simulink model "LeftTurn"  (R2023b)
settings: Solver=FixedStepAuto  StartTime=0.0  StopTime=inf  RelTol=1e-3
undefined symbols (not defined in the file or in its folder): DiscIntNeverNeededParam
libraries: arduinolib x14, simulink x12, mobileRoboticsTrainingLib x1, arduinosensorlib x1
settings Model: ExtModeTrigDuration=2  Creator=cameronclark  LastModifiedBy=cameronclark
settings OptimizationCC: EnhancedBackFolding=on  PassReuseOutputArgsAs=Individual arguments  ZeroExternalMemoryAtStartup=off  ZeroInternalMemoryAtStartup=off  MaxStackSize=64  OptimizeBlockOrder=speed  DifferentSizesBufferReuse=on  OptimizationCustomize=off  EfficientTunableParamExpr=on
settings DebuggingCC: ParameterTunabilityLossMsg=error
settings HardwareCC: ProdBitPerPointer=32  ProdBitPerSizeT=32  ProdBitPerPtrDiffT=32  ProdLargestAtomicInteger=Long  ProdLargestAtomicFloat=Double  ProdWordSize=32  ProdHWDeviceType=ARM Compatible->ARM Cortex  UseEmbeddedCoderFeatures=off  UseSimulinkCoderFeatures=off
settings SFSimCC: MATLABDynamicMemAlloc=off
settings RTWCC: Description=Embedded Coder  SystemTargetFile=ert.tlc  HardwareBoard=Arduino Nano 33 IoT  TemplateMakefile=ert_default_tmf  Toolchain=Arduino ARM  BuildConfiguration=Faster Runs
settings CodeAppCC: ForceParamTrailComments=on  IgnoreCustomStorageClasses=off  OperatorAnnotations=on  SimulinkDataObjDesc=on  SFDataObjDesc=on  InsertBlockDesc=on
settings ERTTargetCC: SupportContinuousTime=on  SupportNonInlinedSFcns=on  SupportVariableSizeSignals=on  ExtModeTransport=3  ExtModeStaticAlloc=on  ExtModeAutomaticAllocSize=off  ExtModeStaticAllocSize=8192  ExtModeMexFile=ext_xcp  ExtModeIntrfLevel=Level2 - Open

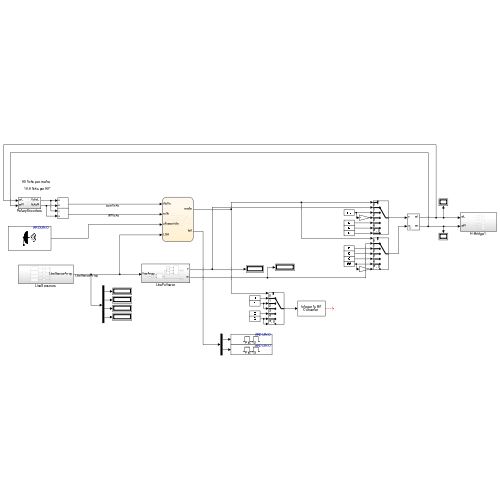
[thumbnail: Simulink's stored preview of the top-level diagram]
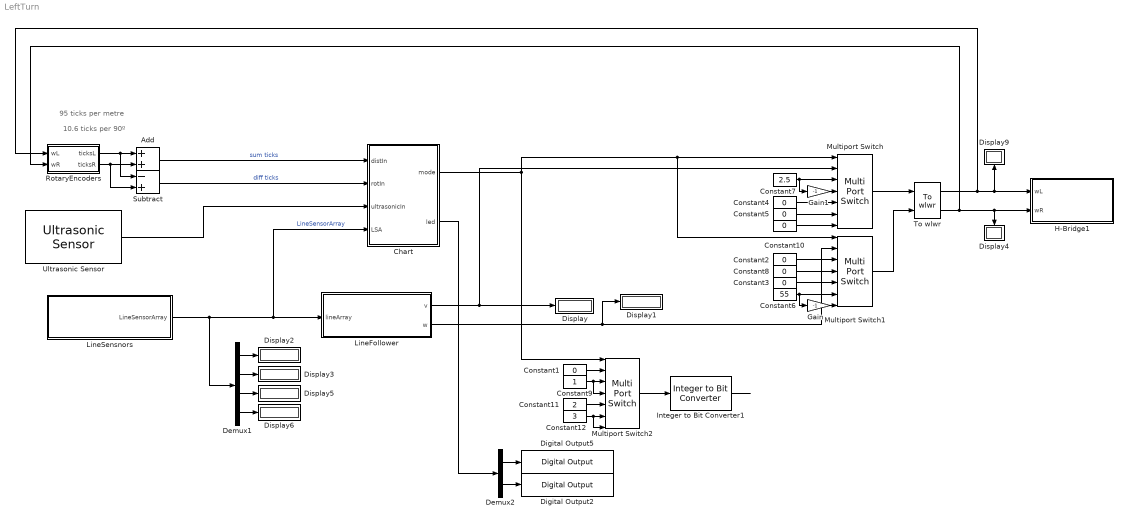
== system LeftTurn ==
  note: 10.6 ticks per 90º
  note: 95 ticks per metre
  Add : Sum
  Chart : Stateflow chart  TreatAsAtomicUnit=on
  Constant{1..5,8,10} (7 alike) : Constant  Value=0
  Constant11 : Constant  Value=2
  Constant12 : Constant  Value=3
  Constant6 : Constant  Value=55
  Constant7 : Constant  Value=2.5
  Constant9 : Constant
  Demux1 : Demux
  Demux2 : Demux  Outputs=2
  Digital Output2 : arduinolib/Digital Output  pinNumber=13  Direction=output  blockPlatform=arduino
  Digital Output5 : arduinolib/Digital Output  pinNumber=12  Direction=output  blockPlatform=arduino
  Display{,1..6,9} (8 alike) : Display
  Gain : Gain  Gain=-1
  Gain1 : Gain  Gain=-1
  H-Bridge1 : Subsystem
  Integer to Bit Converter1 : simulink/Logic and Bit Operations/Integer to Bit Converter  nbits=2  signedInputValues=Unsigned  bitOrder=MSB first  outDtype=Inherit via internal rule
  LineFollower : Subsystem
  LineSensnors : Subsystem
  Multiport Switch : MultiPortSwitch  DataPortOrder=Zero-based contiguous  Inputs=6  DataPortIndices={0,1,3,4}  zeroidx=on  SaturateOnIntegerOverflow=off
  Multiport Switch1 : MultiPortSwitch  DataPortOrder=Zero-based contiguous  Inputs=6  DataPortIndices={0,1,3,4}  zeroidx=on  SaturateOnIntegerOverflow=off  InputSameDT=off
  Multiport Switch2 : MultiPortSwitch  DataPortOrder=Zero-based contiguous  Inputs=6  DataPortIndices={0,1,3,4}  zeroidx=on  SaturateOnIntegerOverflow=off  InputSameDT=off
  RotaryEncoders : Subsystem
  Subtract : Sum  Inputs=-+
  To wlwr : mobileRoboticsTrainingLib/To wlwr  axleLength=0.1  wheelR=0.05
      link override change parameters: Gain=[1 -axleLength/2;1 axleLength/2]
  Ultrasonic Sensor : arduinosensorlib/Ultrasonic Sensor  NumSignalPins=2  TrigPin=8  EchoPin=11  SignalPin=3  SampleTime_=0.1  blockPlatform=ARDUINO
  wires:
  Ultrasonic Sensor/1 -> Chart/3(ultrasonicIn)
  LineFollower/1(v) -> Multiport Switch/2, Display/1
  Multiport Switch/1 -> To wlwr/1
  RotaryEncoders/2(ticksR) -> Subtract/2, Add/2
  Subtract/1 -> Chart/2(rotIn)  "diff ticks"
  Add/1 -> Chart/1(distIn)  "sum ticks"
  Constant7/1 -> Gain1/1, Multiport Switch/3
  LineFollower/2(w) -> Multiport Switch1/2, Display1/1
  RotaryEncoders/1(ticksL) -> Subtract/1, Add/1
  Constant5/1 -> Multiport Switch/6
  Constant2/1 -> Multiport Switch1/3
  Constant3/1 -> Multiport Switch1/5
  Multiport Switch1/1 -> To wlwr/2
  Constant4/1 -> Multiport Switch/5
  LineSensnors/1(LineSensorArray) -> Demux1/1, LineFollower/1(lineArray), Chart/4(LSA)  "LineSensorArray"
  Chart/1(mode) -> Multiport Switch2/1, Multiport Switch1/1, Multiport Switch/1
  Constant8/1 -> Multiport Switch1/4
  Constant10/1 -> Multiport Switch/7
  Demux1/1 -> Display2/1
  Demux1/2 -> Display3/1
  Demux1/3 -> Display5/1
  Demux1/4 -> Display6/1
  To wlwr/2 -> RotaryEncoders/2(wR), H-Bridge1/2(wR), Display4/1
  To wlwr/1 -> RotaryEncoders/1(wL), H-Bridge1/1(wL), Display9/1
  Constant6/1 -> Gain/1, Multiport Switch1/6
  Gain/1 -> Multiport Switch1/7
  Gain1/1 -> Multiport Switch/4
  Integer to Bit Converter1/1 -> ?
  Multiport Switch2/1 -> Integer to Bit Converter1/1
  Constant1/1 -> Multiport Switch2/2
  Constant9/1 -> Multiport Switch2/4, Multiport Switch2/3
  Constant11/1 -> Multiport Switch2/5
  Constant12/1 -> Multiport Switch2/7, Multiport Switch2/6
  Demux2/1 -> Digital Output5/1
  Demux2/2 -> Digital Output2/1
  Chart/2(led) -> Demux2/1

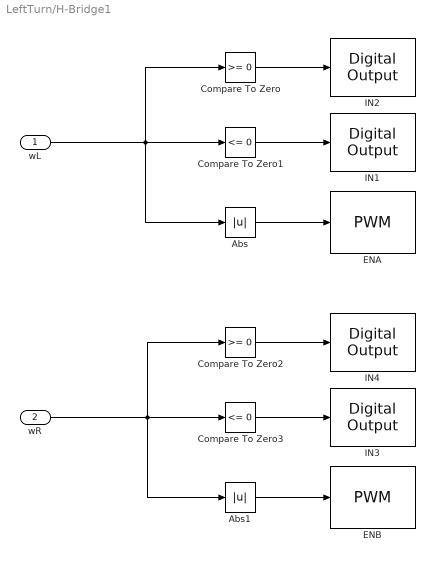
== system LeftTurn/H-Bridge1 ==
  wL : Inport
  wR : Inport  Port=2
  Abs : Abs  SaturateOnIntegerOverflow=off
  Abs1 : Abs  SaturateOnIntegerOverflow=off
  Compare To Zero : simulink/Logic and Bit Operations/Compare To Zero  relop=>=  OutDataTypeStr=boolean
  Compare To Zero1 : simulink/Logic and Bit Operations/Compare To Zero  relop=<=  OutDataTypeStr=boolean
  Compare To Zero2 : simulink/Logic and Bit Operations/Compare To Zero  relop=>=  OutDataTypeStr=boolean
  Compare To Zero3 : simulink/Logic and Bit Operations/Compare To Zero  relop=<=  OutDataTypeStr=boolean
  ENA : arduinolib/PWM  pinNumber=4  frequencyType=Default  desiredFrequency=490.2  achievableFrequency=490.2
  ENB : arduinolib/PWM  pinNumber=5  frequencyType=Default  desiredFrequency=490.2  achievableFrequency=490.2
  IN1 : arduinolib/Digital Output  pinNumber=2  Direction=output  blockPlatform=arduino
  IN2 : arduinolib/Digital Output  pinNumber=3  Direction=output  blockPlatform=arduino
  IN3 : arduinolib/Digital Output  pinNumber=6  Direction=output  blockPlatform=arduino
  IN4 : arduinolib/Digital Output  pinNumber=7  Direction=output  blockPlatform=arduino
  wires:
  Compare To Zero1/1 -> IN1/1
  Compare To Zero/1 -> IN2/1
  Abs1/1 -> ENB/1
  Compare To Zero3/1 -> IN3/1
  Compare To Zero2/1 -> IN4/1
  wL/1 -> Compare To Zero/1, Compare To Zero1/1, Abs/1
  Abs/1 -> ENA/1
  wR/1 -> Compare To Zero2/1, Compare To Zero3/1, Abs1/1

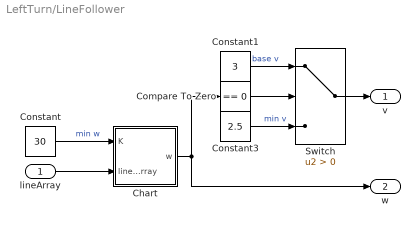
== system LeftTurn/LineFollower ==
  lineArray : Inport
  Chart : Stateflow chart  TreatAsAtomicUnit=on
  Compare To Zero : simulink/Logic and Bit Operations/Compare To Zero  relop===  OutDataTypeStr=boolean
  Constant : Constant  Value=30
  Constant1 : Constant  Value=3
  Constant3 : Constant  Value=2.5
  Switch : Switch  Criteria=u2 > Threshold  SaturateOnIntegerOverflow=off  InputSameDT=off
  v : Outport
  w : Outport  Port=2
  wires:
  Constant1/1 -> Switch/1  "base v"
  Chart/1(w) -> Compare To Zero/1, w/1
  Constant3/1 -> Switch/3  "min v"
  Switch/1 -> v/1
  lineArray/1 -> Chart/2(lineArray)
  Compare To Zero/1 -> Switch/2
  Constant/1 -> Chart/1(K)  "min w"

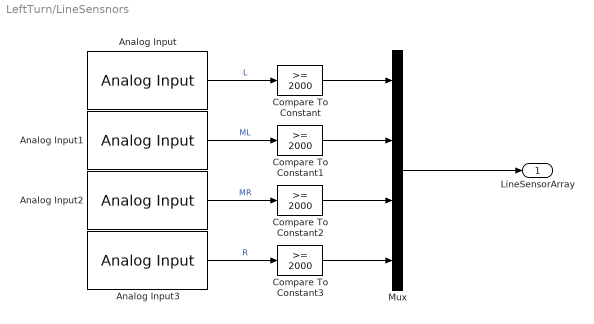
== system LeftTurn/LineSensnors ==
  Analog Input : arduinolib/Analog Input  pinNumber=7  ReadResultsOnly=off  ConversionTriggerSource=Software  ExternalTriggerType=uint32( 0 )  OutputDataType=uint16  EnableConversionCompleteNotify=off  EnableOuputStatus=off  SampleTime=-1  blockPlatform=arduino
  Analog Input1 : arduinolib/Analog Input  pinNumber=6  ReadResultsOnly=off  ConversionTriggerSource=Software  ExternalTriggerType=uint32( 0 )  OutputDataType=uint16  EnableConversionCompleteNotify=off  EnableOuputStatus=off  SampleTime=-1  blockPlatform=arduino
  Analog Input2 : arduinolib/Analog Input  pinNumber=3  ReadResultsOnly=off  ConversionTriggerSource=Software  ExternalTriggerType=uint32( 0 )  OutputDataType=uint16  EnableConversionCompleteNotify=off  EnableOuputStatus=off  SampleTime=-1  blockPlatform=arduino
  Analog Input3 : arduinolib/Analog Input  pinNumber=2  ReadResultsOnly=off  ConversionTriggerSource=Software  ExternalTriggerType=uint32( 0 )  OutputDataType=uint16  EnableConversionCompleteNotify=off  EnableOuputStatus=off  SampleTime=-1  blockPlatform=arduino
  Compare To Constant{,1..3} (4 alike) : simulink/Logic and Bit Operations/Compare To Constant  relop=>=  const=2000  OutDataTypeStr=boolean
  Mux : Mux
  LineSensorArray : Outport
  wires:
  Mux/1 -> LineSensorArray/1
  Analog Input/1 -> Compare To Constant/1  "L"
  Analog Input1/1 -> Compare To Constant1/1  "ML"
  Analog Input2/1 -> Compare To Constant2/1  "MR"
  Analog Input3/1 -> Compare To Constant3/1  "R"
  Compare To Constant/1 -> Mux/1
  Compare To Constant1/1 -> Mux/2
  Compare To Constant2/1 -> Mux/3
  Compare To Constant3/1 -> Mux/4

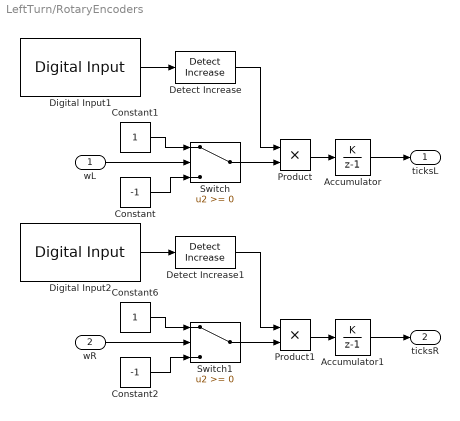
== system LeftTurn/RotaryEncoders ==
  wL : Inport
  wR : Inport  Port=2
  Accumulator : DiscreteIntegrator  IntegratorMethod=Accumulation: Forward Euler  SampleTime=-1  ICPrevOutput=DiscIntNeverNeededParam  ICPrevScaledInput=DiscIntNeverNeededParam
  Accumulator1 : DiscreteIntegrator  IntegratorMethod=Accumulation: Forward Euler  SampleTime=-1  ICPrevOutput=DiscIntNeverNeededParam  ICPrevScaledInput=DiscIntNeverNeededParam
  Constant : Constant  Value=-1
  Constant1 : Constant
  Constant2 : Constant  Value=-1
  Constant6 : Constant
  Detect Increase : simulink/Logic and Bit Operations/Detect Increase  vinit=0.0  OutDataTypeStr=boolean
  Detect Increase1 : simulink/Logic and Bit Operations/Detect Increase  vinit=0.0  OutDataTypeStr=boolean
  Digital Input1 : arduinolib/Digital Input  pinNumber=9  mode=Default  Direction=input  SampleTime=0.1  blockPlatform=arduino
  Digital Input2 : arduinolib/Digital Input  pinNumber=10  mode=Default  Direction=input  SampleTime=0.1  blockPlatform=arduino
  Product : Product
  Product1 : Product
  Switch : Switch  SaturateOnIntegerOverflow=off  InputSameDT=off
  Switch1 : Switch  SaturateOnIntegerOverflow=off  InputSameDT=off
  ticksL : Outport
  ticksR : Outport  Port=2
  wires:
  wL/1 -> Switch/2
  Constant1/1 -> Switch/1
  Constant/1 -> Switch/3
  Digital Input1/1 -> Detect Increase/1
  Switch/1 -> Product/2
  Accumulator/1 -> ticksL/1
  wR/1 -> Switch1/2
  Constant6/1 -> Switch1/1
  Constant2/1 -> Switch1/3
  Accumulator1/1 -> ticksR/1
  Switch1/1 -> Product1/2
  Product/1 -> Accumulator/1
  Detect Increase/1 -> Product/1
  Detect Increase1/1 -> Product1/1
  Digital Input2/1 -> Detect Increase1/1
  Product1/1 -> Accumulator1/1

== stateflow chart LeftTurn/LineFollower/Chart ==
  state ComputeW
    %code for the line array
    during:
    w = K*(lineArray(3)-lineArray(2));
  (default) -> ComputeW
  data: w output; K input; lineArray input

== stateflow chart LeftTurn/Chart ==
  state Setup
    entry:
    stop=0;
    objects = ones(5);
    object = 1;
  state Drive
    entry:
    mode=0;
    led = [false false];
  state TurnToLine
    entry:
    mode = 4;
  state Stop
    entry:
    mode=3;
  state DriveAway
    entry:
    mode = 0;
    distT = distIn + 6;
  state DriveBackward1
    entry:
    mode = 2;
  state Party
    state dance
      entry:
      moves = moves + 1;
    dance -> (junction 71) [order 2] : {mode=1;}
        | %1
    (junction 101) -> dance
    (junction 97) -> (junction 101) : after(125, msec)
    (junction 71) -> (junction 73) : after(250, msec)
        | {mode=2;}
        | %1+
    (junction 98) -> (junction 97) : after(125, msec)
        | {mode=3;}
        | %4a+d
    (junction 73) -> (junction 75) : after(250, msec)
        | {mode=4;}
        | %2
    (junction 75) -> (junction 76) : after(250, msec)
        | {mode=5;}
        | %2a+
    (junction 90) -> (junction 98) : after(250, msec)
        | {mode=5;}
        | %4a+
    (junction 76) -> (junction 77) : after(125, msec)
        | {mode=3;}
        | %2a+d
    (junction 85) -> (junction 90) : after(125, msec)
        | {mode=4;}
        | %4
    (junction 77) -> (junction 81) : after(125, msec)
        | {mode=4;}
        | %3
    (junction 81) -> (junction 91) : after(250, msec)
        | {mode=5;}
        | %3a+
    (junction 91) -> (junction 85) : after(125, msec)
        | {mode=3;}
        | %3a+d
  state DriveForward
    entry:
    mode = 1;
    distT = distIn + 4;
  state CentreOnIntersection
    entry:
    mode = 1;
    distT = distIn + 5;
  state LeftTurn
    entry:
    mode = 4;
    rotT = rotIn + 13;
  state RightTurn
    entry:
    mode = 5;
  state CentreOnIntersection1
    entry:
    mode = 1;
    distT = distIn + 5;
  state TurnAround
    entry:
    mode = 4;
    rotT = rotIn + 14;
  state ErrorHandler
    entry:
    mode=4;
  state ClosestObject
    entry:
    cObj = 1;
    for i = 1:5
    if objects(i) < cObj
    cObj = objects(i);
    end
    end
  state DriveBackward
    entry:
    mode = 2;
  state USmeasure
    entry:
    led = [(ultrasonicIn < 0.1) (ultrasonicIn < 0.2)] ;
    objects(object) = ultrasonicIn;
    object = object + 1;
  state Pause
    entry:
    mode=3;
    moves = 0;
  (default) -> Setup
  Setup -> Drive
  Drive -> TurnToLine [order 1] : [all(LSA==1)]
  TurnToLine -> DriveBackward1 : [LSA(2)==0]
  Drive -> CentreOnIntersection [order 2] : [~LSA(1) | ~LSA(4)]{mode=3;}
  DriveAway -> Drive : [distIn>distT]
  dance -> Stop [order 1] : [moves > 4]
  DriveBackward1 -> DriveAway : [LSA(2)==1 | LSA(3)==1]
  RightTurn -> DriveAway : [LSA(2)==0]
  TurnAround -> DriveAway : [rotIn>rotT & LSA(3)==0]
  Pause -> (junction 71) : after(3,sec)
      | {mode=1;}
      | %1
  CentreOnIntersection -> LeftTurn [order 2] : [distIn>distT]
  CentreOnIntersection -> DriveForward [order 1] : [~LSA(1) & ~LSA(4)]
  LeftTurn -> RightTurn : [rotIn>rotT]
  DriveForward -> DriveBackward [order 1] : [LSA(1) & LSA(4)]
  CentreOnIntersection1 -> LeftTurn : [distIn>distT]
  DriveForward -> (junction 35) [order 2] : [distIn>distT]
      | {stop = stop + 1;}
  (junction 54) -> CentreOnIntersection1 [order 2]
  (junction 35) -> ErrorHandler [order 2] : [stop>2]
  (junction 35) -> (junction 63) [order 3]
  (junction 63) -> TurnAround
  (junction 57) -> (junction 63) [order 2]
  ClosestObject -> (junction 63)
  (junction 141) -> (junction 63) [order 1] : [stop==0]
  (junction 35) -> ClosestObject [order 1] : [stop==2]
  USmeasure -> (junction 63)
  DriveBackward -> (junction 54) : [~LSA(1) & ~LSA(4)]
      | {mode=3}
  (junction 54) -> (junction 141) [order 1] : [ultrasonicIn & (ultrasonicIn < 0.5)]
  (junction 141) -> USmeasure [order 3]
  (junction 141) -> (junction 57) [order 2] : [stop==2]
  (junction 57) -> Pause [order 1] : [abs(ultrasonicIn-cObj) <= 0.03]
  data: distIn input; rotIn input; mode output; ultrasonicIn input; LSA input; distT local; rotT local; objects local; stop local; cObj local; i local; object local; moves local; led output
